simulink model "simulazioneAnticipo"  (R2020a)
settings: Solver=FixedStepDiscrete  StartTime=0.0  StopTime=40.0  FixedStep=1  RelTol=1e-3
settings Model: Creator=aless  LastModifiedBy=aless

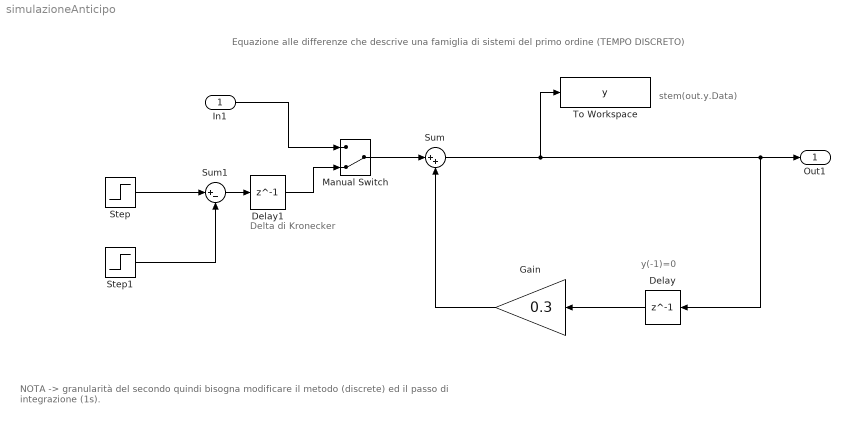
== system simulazioneAnticipo ==
  note: stem(out.y.Data)
  note: y(-1)=0
  note: NOTA -> granularità del secondo quindi bisogna modificare il metodo (discrete) ed il passo di integrazione (1s).
  note: Equazione alle differenze che descrive una famiglia di sistemi del primo ordine (TEMPO DISCRETO)
  note: Delta di Kronecker
  In1 : Inport
  Delay : Delay  DelayLength=1  InitialCondition=0
  Delay1 : Delay  DelayLength=1  InitialCondition=0
  Gain : Gain  Gain=0.3
  Manual Switch : ManualSwitch  CurrentSetting=0
  Step : Step  Time=0  SampleTime=0
  Step1 : Step  SampleTime=0
  Sum : Sum  Inputs=|++
  Sum1 : Sum  Inputs=|+-
  To Workspace : ToWorkspace  VariableName=y  SaveFormat=Timeseries  SampleTime=-1
  Out1 : Outport
  wires:
  Sum/1 -> To Workspace/1, Delay/1, Out1/1
  Gain/1 -> Sum/2
  Delay/1 -> Gain/1
  Manual Switch/1 -> Sum/1
  In1/1 -> Manual Switch/1
  Step/1 -> Sum1/1
  Step1/1 -> Sum1/2
  Sum1/1 -> Delay1/1
  Delay1/1 -> Manual Switch/2
